simulink model "dynamic_range_compression_sim"  (R2020b)
settings: Solver=FixedStepAuto  StartTime=0.0  StopTime=stop_time  RelTol=1e-3
InitFcn:
  | dynamic_range_compression_sim_init
StopFcn:
  | dynamic_range_compression_sim_stop
values from neighbouring files (symbols this model uses):
  fs = audio_fs * fft_up_sample_rate    (= 6144000)    [dynamic_range_compression_sim_init.m]    (also in test_FFT_to_gain_init.m = 48000)
settings Model: SnapshotBufferSize=20  Creator=t96f346  LastModifiedBy=conno
settings SolverCC: AutoInsertRateTranBlk=on
settings DataIOCC: ReturnWorkspaceOutputs=off
settings HardwareCC: ProdBitPerPointer=32  ProdBitPerSizeT=32  ProdBitPerPtrDiffT=32  ProdLargestAtomicFloat=None  ProdWordSize=32  ProdHWDeviceType=Altera->SoC (ARM Cortex A)

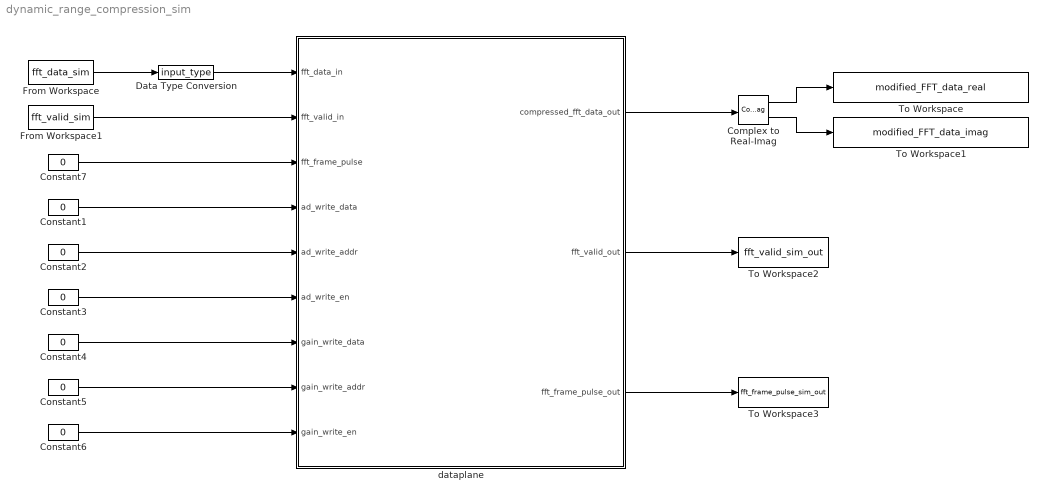
== system dynamic_range_compression_sim ==
  Complex to Real-Imag : ComplexToRealImag
  Constant1 : Constant  Value=0  OutDataTypeStr=ad_coeff_type  SampleTime=-1
  Constant2 : Constant  Value=0  OutDataTypeStr=uint8  SampleTime=-1
  Constant3 : Constant  Value=0  OutDataTypeStr=boolean  SampleTime=-1
  Constant4 : Constant  Value=0  OutDataTypeStr=gain_coeff_type  SampleTime=-1
  Constant5 : Constant  Value=0  OutDataTypeStr=uint8  SampleTime=-1
  Constant6 : Constant  Value=0  OutDataTypeStr=boolean  SampleTime=-1
  Constant7 : Constant  Value=0  OutDataTypeStr=boolean  SampleTime=-1
  Data Type Conversion : DataTypeConversion  OutDataTypeStr=input_type
  From Workspace : FromWorkspace  VariableName=fft_data_sim  SampleTime=-1  Interpolate=off  OutputAfterFinalValue=Holding final value
  From Workspace1 : FromWorkspace  VariableName=fft_valid_sim  SampleTime=1/fs
  To Workspace : ToWorkspace  VariableName=modified_FFT_data_real  SampleTime=-1
      settings: Save2DSignal=2-D array (concatenate along first dimension)
  To Workspace1 : ToWorkspace  VariableName=modified_FFT_data_imag  SampleTime=-1
      settings: Save2DSignal=2-D array (concatenate along first dimension)
  To Workspace2 : ToWorkspace  VariableName=fft_valid_sim_out  SampleTime=-1
  To Workspace3 : ToWorkspace  VariableName=fft_frame_pulse_sim_out  SampleTime=-1
  dataplane : Subsystem
  wires:
  Complex to Real-Imag/2 -> To Workspace1/1
  Complex to Real-Imag/1 -> To Workspace/1
  dataplane/1("compressed_fft_data_out ") -> Complex to Real-Imag/1
  dataplane/2("fft_valid_out ") -> To Workspace2/1
  dataplane/3(fft_frame_pulse_out) -> To Workspace3/1
  From Workspace/1 -> Data Type Conversion/1
  From Workspace1/1 -> dataplane/2(fft_valid_in)
  Constant7/1 -> dataplane/3(fft_frame_pulse)
  Constant1/1 -> dataplane/4(ad_write_data)
  Constant2/1 -> dataplane/5(ad_write_addr)
  Constant3/1 -> dataplane/6(ad_write_en)
  Constant4/1 -> dataplane/7(gain_write_data)
  Constant6/1 -> dataplane/9(gain_write_en)
  Constant5/1 -> dataplane/8(gain_write_addr)
  Data Type Conversion/1 -> dataplane/1(fft_data_in)

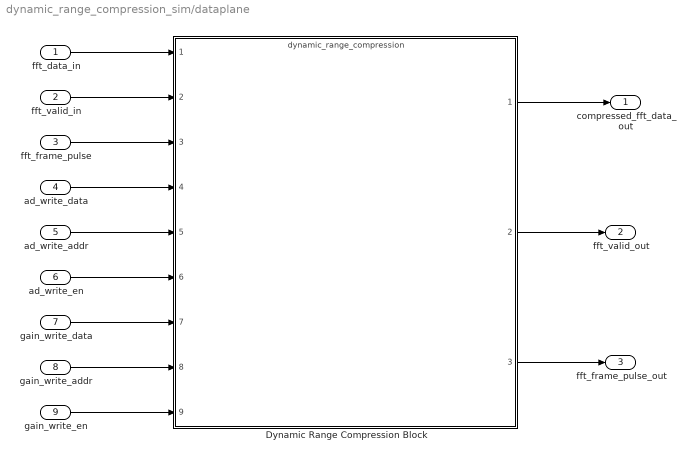
== system dynamic_range_compression_sim/dataplane ==
  fft_data_in : Inport
  fft_valid_in : Inport  Port=2
  fft_frame_pulse : Inport  Port=3
  ad_write_data : Inport  Port=4
  ad_write_addr : Inport  Port=5
  ad_write_en : Inport  Port=6
  gain_write_data : Inport  Port=7
  gain_write_addr : Inport  Port=8
  gain_write_en : Inport  Port=9
  Dynamic Range Compression Block : ModelReference  ModelNameDialog=dynamic_range_compression  SimulationMode=Normal  ModelReferenceVersion=2.69
  "compressed_fft_data_out " : Outport
  "fft_valid_out " : Outport  Port=2
  fft_frame_pulse_out : Outport  Port=3
  wires:
  gain_write_en/1 -> Dynamic Range Compression Block/9
  gain_write_addr/1 -> Dynamic Range Compression Block/8
  gain_write_data/1 -> Dynamic Range Compression Block/7
  ad_write_en/1 -> Dynamic Range Compression Block/6
  ad_write_addr/1 -> Dynamic Range Compression Block/5
  ad_write_data/1 -> Dynamic Range Compression Block/4
  fft_frame_pulse/1 -> Dynamic Range Compression Block/3
  fft_valid_in/1 -> Dynamic Range Compression Block/2
  fft_data_in/1 -> Dynamic Range Compression Block/1
  Dynamic Range Compression Block/1 -> "compressed_fft_data_out "/1
  Dynamic Range Compression Block/2 -> "fft_valid_out "/1
  Dynamic Range Compression Block/3 -> fft_frame_pulse_out/1
